simulink model "Digiral Controller"  (R2019a)
settings: Solver=VariableStepAuto  StartTime=0.0  StopTime=2000.0  RelTol=1e-3
settings Model: Creator=atefeh  LastModifiedBy=atefeh

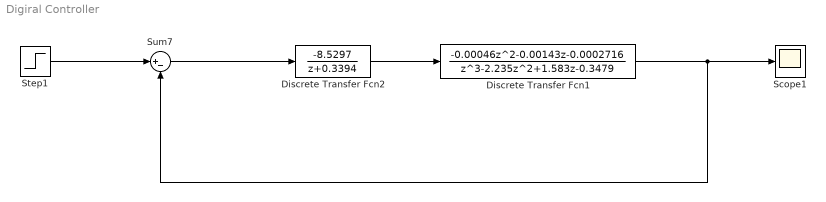
== system Digiral Controller ==
  "Discrete Transfer Fcn1 " : DiscreteTransferFcn  Numerator=[-0.00046 -0.00143 -0.0002716]  Denominator=[1 -2.235 1.583 -0.3479]  SampleTime=9
  "Discrete Transfer Fcn2 " : DiscreteTransferFcn  Numerator=[-8.5297]  Denominator=[1 0.3394]  SampleTime=9
  "Scope1 " : Scope
  "Step1 " : Step  SampleTime=0
  Sum7 : Sum  Inputs=|+-
  wires:
  Sum7/1 -> "Discrete Transfer Fcn2 "/1
  "Discrete Transfer Fcn1 "/1 -> Sum7/2, "Scope1 "/1
  "Step1 "/1 -> Sum7/1
  "Discrete Transfer Fcn2 "/1 -> "Discrete Transfer Fcn1 "/1
